simulink model "SimpleNeuronTest"  (Simulink 9.2)
settings: Solver=ode45  StartTime=0.0  StopTime=10.0  RelTol=1e-3  EnableMultiTasking=on
libraries: NeuroModelerLibrary x7
settings Model: Creator=Tim  LastModifiedBy=Bakhshiev
settings DataIOCC: SignalLoggingSaveFormat=Dataset
settings DebuggingCC: UnderspecifiedInitializationDetection=Simplified  MergeDetectMultiDrivingBlocksExec=error  SolverPrmCheckMsg=warning  FcnCallInpInsideContextMsg=error  StateNameClashWarn=none
settings GRTTargetCC: CombineOutputUpdateFcns=on  GRTInterface=off
settings ConfigComp: CovSFcnEnable=off

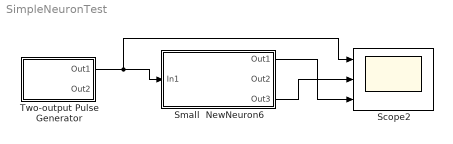
== system SimpleNeuronTest ==
  Scope2 : Scope  NumInputPorts=3
  Small  NewNeuron6 : Subsystem
  Two-output Pulse Generator : Subsystem  mask{A=100, P1=400, P2=100, PW=1, ST=0.001, OOn1=0.04, OOff1=0.5, OOn2=0.4, OOff2=20}
      mask prompts: A "Amplitude"; P1 "Out1: Period (number of samples)"; P2 "Out2: Period (number of samples)"; PW "Pulse Width (number of samples)"; ST "Sample Time"; OOn1 "Out1 On (seconds)"; OOff1 "Out1 Off (seconds)"; OOn2 "Out2 On (seconds)"; OOff2 "Out2 Off (seconds)"
  wires:
  Two-output Pulse Generator/1(Out1) -> Small  NewNeuron6/1(In1), Scope2/1
  Small  NewNeuron6/1(Out1) -> Scope2/3
  Small  NewNeuron6/3(Out3) -> Scope2/2

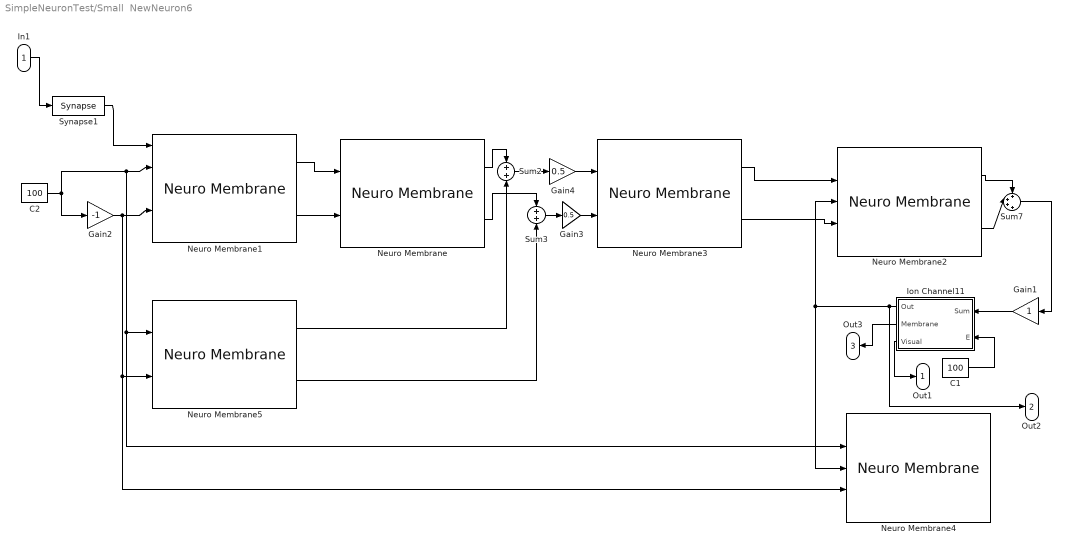
== system SimpleNeuronTest/Small  NewNeuron6 ==
  In1 : Inport
  C1 : Constant  Value=100
  C2 : Constant  Value=100
  Gain1 : Gain  OutDataTypeStr=Inherit: Same as input  ParamDataTypeStr=Inherit: Same as input
  Gain2 : Gain  Gain=-1  OutDataTypeStr=Inherit: Same as input  ParamDataTypeStr=Inherit: Same as input
  Gain3 : Gain  Gain=0.5  OutDataTypeStr=Inherit: Same as input  ParamDataTypeStr=Inherit: Same as input
  Gain4 : Gain  Gain=0.5  OutDataTypeStr=Inherit: Same as input  ParamDataTypeStr=Inherit: Same as input
  Ion Channel11 : Subsystem  mask(Ion pump){Rc=1, Cc=0.001, RR=1, IT=0.005, T=10}
      mask prompts: Rc "Channel resistance"; Cc "Channel capacity"; RR "Recharge Resistance"; IT "Input TC"; T "Threshold"
  Neuro Membrane{,1..5} (6 alike) : NeuroModelerLibrary/Old Neuron Elements/Neuro Membrane  ACm=0.1  ARm=1  ECm=0.1  ERm=1
  Sum2 : Sum  SaturateOnIntegerOverflow=on  InputSameDT=on  OutDataTypeStr=Inherit: Same as first input
  Sum3 : Sum  SaturateOnIntegerOverflow=on  InputSameDT=on  OutDataTypeStr=Inherit: Same as first input
  Sum7 : Sum  Inputs=++++  SaturateOnIntegerOverflow=on  InputSameDT=on  OutDataTypeStr=Inherit: Same as first input
  Synapse1 : NeuroModelerLibrary/Old Neuron Elements/Synapse  SecretionTC=0.001  DecompositionTC=0.1  ksi=1  gamma=1
  Out1 : Outport
  Out2 : Outport  Port=2
  Out3 : Outport  Port=3
  wires:
  C2/1 -> Neuro Membrane1/2, Neuro Membrane4/2, Neuro Membrane5/2, Gain2/1
  Gain2/1 -> Neuro Membrane1/4, Neuro Membrane4/4, Neuro Membrane5/4
  Neuro Membrane2/2 -> Sum7/2
  Sum7/1 -> Gain1/1
  Neuro Membrane2/1 -> Sum7/1
  C1/1 -> Ion Channel11/2(E)
  In1/1 -> Synapse1/1
  Synapse1/1 -> Neuro Membrane1/1
  Ion Channel11/1(Out) -> Out2/1, Neuro Membrane4/3, Neuro Membrane2/3
  Neuro Membrane1/1 -> Neuro Membrane/2
  Neuro Membrane1/2 -> Neuro Membrane/4
  Neuro Membrane3/1 -> Neuro Membrane2/2
  Neuro Membrane3/2 -> Neuro Membrane2/4
  Neuro Membrane/1 -> Sum2/1
  Neuro Membrane/2 -> Sum3/1
  Sum3/1 -> Gain3/1
  Sum2/1 -> Gain4/1
  Neuro Membrane5/1 -> Sum2/2
  Neuro Membrane5/2 -> Sum3/2
  Gain1/1 -> Ion Channel11/1(Sum)
  Ion Channel11/3(Visual) -> Out1/1
  Gain3/1 -> Neuro Membrane3/4
  Gain4/1 -> Neuro Membrane3/2
  Ion Channel11/2(Membrane) -> Out3/1

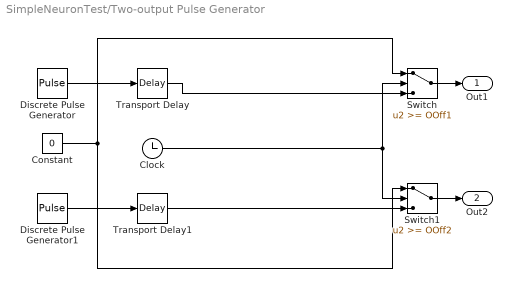
== system SimpleNeuronTest/Two-output Pulse Generator ==
  Clock : Clock
  Constant : Constant  Value=0
  Discrete Pulse Generator : DiscretePulseGenerator  Amplitude=A  Period=P1  PulseWidth=PW  SampleTime=ST
  Discrete Pulse Generator1 : DiscretePulseGenerator  Amplitude=A  Period=P2  PulseWidth=PW  SampleTime=ST
  Switch : Switch  Threshold=OOff1  SaturateOnIntegerOverflow=on  InputSameDT=on
  Switch1 : Switch  Threshold=OOff2  SaturateOnIntegerOverflow=on  InputSameDT=on
  Transport Delay : TransportDelay  DelayTime=OOn1
  Transport Delay1 : TransportDelay  DelayTime=OOn2
  Out1 : Outport  InitialOutput=0
  Out2 : Outport  Port=2  InitialOutput=0
  wires:
  Discrete Pulse Generator/1 -> Transport Delay/1
  Constant/1 -> Switch/1, Switch1/1
  Discrete Pulse Generator1/1 -> Transport Delay1/1
  Transport Delay1/1 -> Switch1/3
  Transport Delay/1 -> Switch/3
  Clock/1 -> Switch/2, Switch1/2
  Switch/1 -> Out1/1
  Switch1/1 -> Out2/1

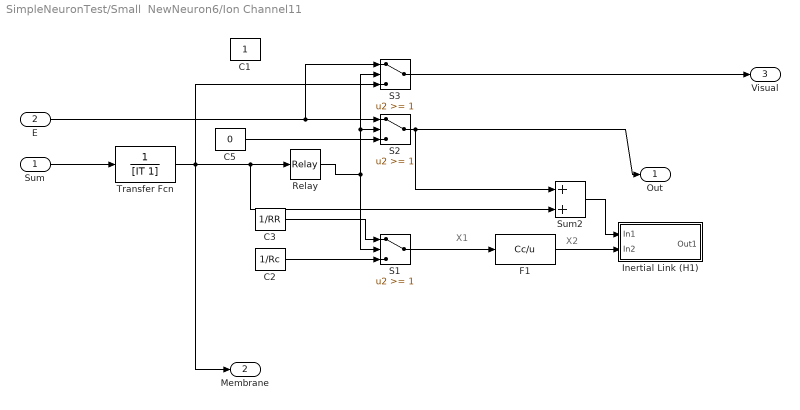
== system SimpleNeuronTest/Small  NewNeuron6/Ion Channel11 ==
  note: X2
  note: X1
  Sum : Inport
  E : Inport  Port=2
  C1 : Constant
  C2 : Constant  Value=1/Rc
  C3 : Constant  Value=1/RR
  C5 : Constant  Value=0
  F1 : Fcn  Expr=Cc/u
  Inertial Link (H1) : Subsystem
  Relay : Relay  OnSwitchValue=T  OffSwitchValue=0
  S1 : Switch  Threshold=1  SaturateOnIntegerOverflow=on  InputSameDT=on
  S2 : Switch  Threshold=1  SaturateOnIntegerOverflow=on  InputSameDT=on
  S3 : Switch  Threshold=1  SaturateOnIntegerOverflow=on  InputSameDT=on
  Sum2 : Sum  SaturateOnIntegerOverflow=on  InputSameDT=on  OutDataTypeStr=Inherit: Same as first input
  Transfer Fcn : TransferFcn  Denominator=[IT 1]
  Out : Outport  InitialOutput=0
  Membrane : Outport  Port=2  InitialOutput=0
  Visual : Outport  Port=3  InitialOutput=0
  wires:
  Sum2/1 -> Inertial Link (H1)/1(In1)
  F1/1 -> Inertial Link (H1)/2(In2)
  C2/1 -> S1/3
  C3/1 -> S1/1
  Sum/1 -> Transfer Fcn/1
  C5/1 -> S2/3
  E/1 -> S2/1, S3/1
  S2/1 -> Sum2/1, Out/1
  S1/1 -> F1/1
  Transfer Fcn/1 -> Sum2/2, Relay/1, S3/3, Membrane/1
  Relay/1 -> S1/2, S2/2, S3/2
  S3/1 -> Visual/1

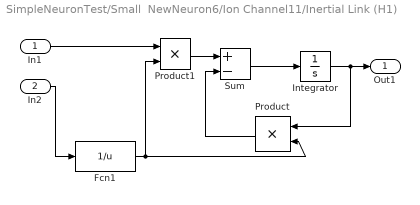
== system SimpleNeuronTest/Small  NewNeuron6/Ion Channel11/Inertial Link (H1) ==
  In1 : Inport
  In2 : Inport  Port=2
  Fcn1 : Fcn  Expr=1/u
  Integrator : Integrator
  Product : Product  SaturateOnIntegerOverflow=on  RndMeth=Zero  InputSameDT=on  OutDataTypeStr=Inherit: Same as first input
  Product1 : Product  SaturateOnIntegerOverflow=on  RndMeth=Zero  InputSameDT=on  OutDataTypeStr=Inherit: Same as first input
  Sum : Sum  Inputs=+-  SaturateOnIntegerOverflow=on  InputSameDT=on  OutDataTypeStr=Inherit: Same as first input
  Out1 : Outport  InitialOutput=0
  wires:
  Sum/1 -> Integrator/1
  Product/1 -> Sum/2
  Product1/1 -> Sum/1
  Fcn1/1 -> Product/2, Product1/2
  Integrator/1 -> Product/1, Out1/1
  In1/1 -> Product1/1
  In2/1 -> Fcn1/1
